simulink model "lane_following_AMPC"  (R2018b)
settings: Solver=VariableStepAuto  StartTime=0.0  StopTime=Duration  RelTol=1e-3
undefined symbols (not defined in the file or in its folder): Cf, Cr, Iz, lf, lr, m, rho, tau, Ts, v0, v_set
libraries: mpclib x1
settings Model: Creator=alberto  LastModifiedBy=alberto

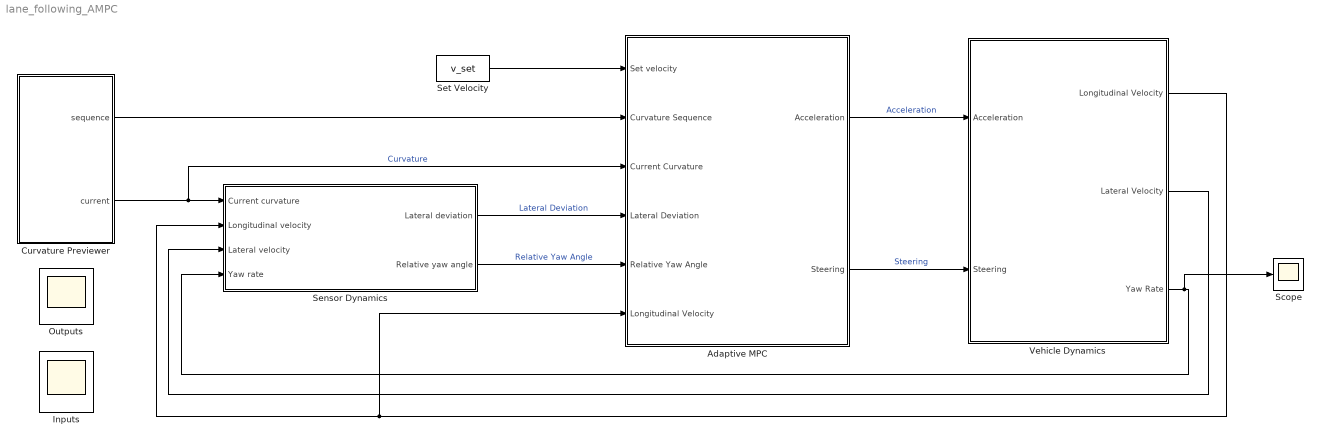
== system lane_following_AMPC ==
  Adaptive MPC : Subsystem  VariantControl=controller_type == 2
  Curvature Previewer : Subsystem  mask{signal=rho, ts=Ts, steps=25}
      mask prompts: signal "Signal name"; ts "Sampling time"; steps "Number of previewing steps"
      mask init:
      | ts = evalin('base',get_param(gcbh,'ts'));
      | signal = evalin('base',get_param(gcbh,'signal'));
      | steps = evalin('base',get_param(gcbh,'steps'));
      | data = mpc_previewer_maskinit(signal,ts);
      mask Display:
      | fprintf('Future\nsample\nextractor');
      | port_label('output', 1, 'seq')
      | port_label('output', 2, '@t')
  Inputs : Scope
      settings: Floating=on
  Outputs : Scope
      settings: Floating=on
  Scope : Scope
  Sensor Dynamics : Subsystem
  Set Velocity : Constant  Value=v_set
  Vehicle Dynamics : Subsystem
  wires:
  Curvature Previewer/2(current) -> Adaptive MPC/3(Current Curvature), Sensor Dynamics/1(Current curvature)  "Curvature"
  Sensor Dynamics/1(Lateral deviation) -> Adaptive MPC/4(Lateral Deviation)  "Lateral Deviation"
  Curvature Previewer/1(sequence) -> Adaptive MPC/2(Curvature Sequence)
  Sensor Dynamics/2(Relative yaw angle) -> Adaptive MPC/5(Relative Yaw Angle)  "Relative Yaw Angle"
  Adaptive MPC/2(" Steering") -> Vehicle Dynamics/2(Steering)  "Steering"
  Set Velocity/1 -> Adaptive MPC/1(Set velocity)
  Adaptive MPC/1(Acceleration) -> Vehicle Dynamics/1(Acceleration)  "Acceleration"
  Vehicle Dynamics/2(Lateral Velocity) -> Sensor Dynamics/3(Lateral velocity)
  Vehicle Dynamics/3(Yaw Rate) -> Scope/1, Sensor Dynamics/4(Yaw rate)
  Vehicle Dynamics/1(Longitudinal Velocity) -> Sensor Dynamics/2(Longitudinal velocity), Adaptive MPC/6(Longitudinal Velocity)

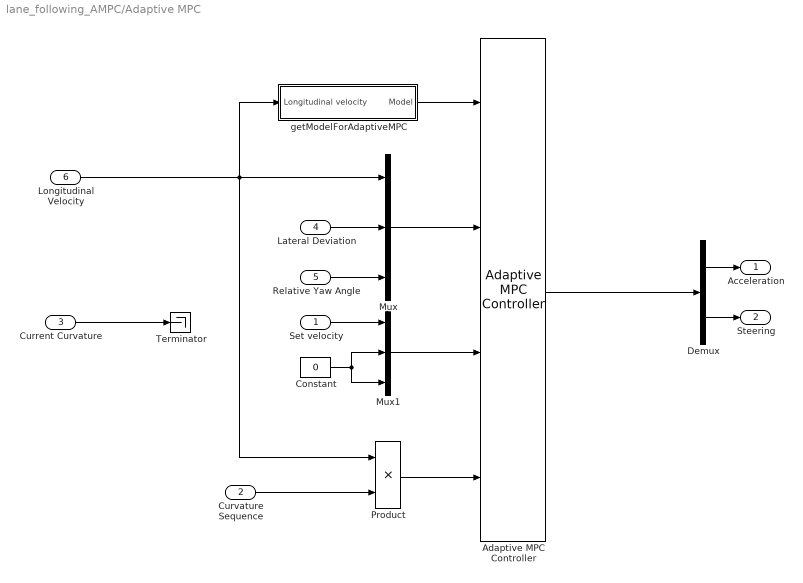
== system lane_following_AMPC/Adaptive MPC ==
  Set velocity : Inport
  Curvature Sequence : Inport  Port=2
  Current Curvature : Inport  Port=3
  Lateral Deviation : Inport  Port=4
  Relative Yaw Angle : Inport  Port=5
  Longitudinal Velocity : Inport  Port=6
  Adaptive MPC Controller : mpclib/Adaptive MPC Controller  SCDEnableBlockLinearizationSpecification=on  mpcobj=mpc1  enable_value=0  updateMPCinCallerWorkspace=on  md_inport=on  mv_inport=off  return_cost=off  return_mvseq=off  return_qpstatus=off  return_xseq=off  return_state=off  return_ovseq=off  state_inport=off  isltv_plant=off  umin_inport=off  umax_inport=off  ymin_inport=off  ymax_inport=off  cc_inport=off  ywt_inport=off  uwt_inport=off  duwt_inport=off  rhoeps_inport=off  uref_inport=off  BlockDataType=double  SampleTimeInherited=off  switch_inport=off
      settings: SourceProductName=Model Predictive Control Toolbox
  Constant : Constant  Value=0
  Demux : Demux  Outputs=2
  Mux : Mux  Inputs=3
  Mux1 : Mux  Inputs=3
  Product : Product
  Terminator : Terminator
  getModelForAdaptiveMPC : Subsystem
  Acceleration : Outport
  " Steering" : Outport  Port=2
  wires:
  Lateral Deviation/1 -> Mux/2
  Longitudinal Velocity/1 -> Product/1, Mux/1, getModelForAdaptiveMPC/1(Longitudinal velocity)
  Relative Yaw Angle/1 -> Mux/3
  Demux/2 -> " Steering"/1
  Set velocity/1 -> Mux1/1
  Demux/1 -> Acceleration/1
  Mux/1 -> Adaptive MPC Controller/2
  Mux1/1 -> Adaptive MPC Controller/3
  Constant/1 -> Mux1/3, Mux1/2
  Product/1 -> Adaptive MPC Controller/4
  getModelForAdaptiveMPC/1(Model) -> Adaptive MPC Controller/1
  Curvature Sequence/1 -> Product/2
  Current Curvature/1 -> Terminator/1
  Adaptive MPC Controller/1 -> Demux/1

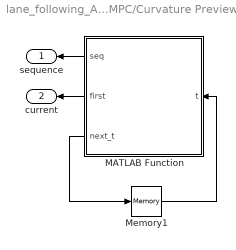
== system lane_following_AMPC/Curvature Previewer ==
  MATLAB Function : MATLAB Function  TreatAsAtomicUnit=on
  Memory1 : Memory  InheritSampleTime=on  LinearizeAsDelay=on
  sequence : Outport
  current : Outport  Port=2
  wires:
  MATLAB Function/1(seq) -> sequence/1
  MATLAB Function/2(first) -> current/1
  Memory1/1 -> MATLAB Function/1(t)
  MATLAB Function/3(next_t) -> Memory1/1

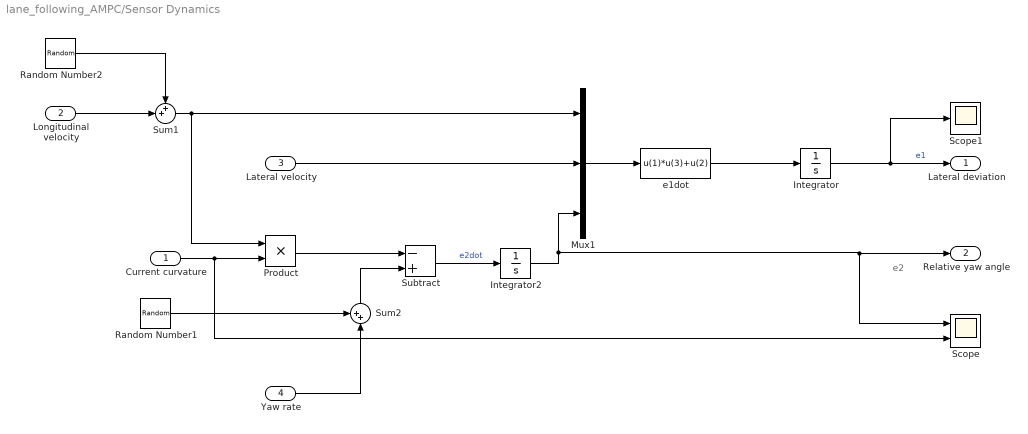
== system lane_following_AMPC/Sensor Dynamics ==
  note: e2
  Current curvature : Inport
  Longitudinal velocity : Inport  Port=2
  Lateral velocity : Inport  Port=3
  Yaw rate : Inport  Port=4
  Integrator : Integrator
  Integrator2 : Integrator
  Mux1 : Mux  Inputs=[1 1 1]
  Product : Product
  Random Number1 : RandomNumber  Variance=0.0003  SampleTime=Ts
  Random Number2 : RandomNumber  Variance=0.3  SampleTime=Ts
  Scope : Scope  NumInputPorts=2
  Scope1 : Scope
  Subtract : Sum  Inputs=-+
  Sum1 : Sum  Inputs=++|
  Sum2 : Sum  Inputs=++|
  e1dot : Fcn  Expr=u(1)*u(3)+u(2)
  Lateral deviation : Outport
  Relative yaw angle : Outport  Port=2
  wires:
  Mux1/1 -> e1dot/1
  Lateral velocity/1 -> Mux1/2
  Product/1 -> Subtract/1
  Subtract/1 -> Integrator2/1  "e2dot"
  Current curvature/1 -> Scope/2, Product/2
  Integrator/1 -> Scope1/1, Lateral deviation/1  "e1"
  Integrator2/1 -> Scope/1, Relative yaw angle/1, Mux1/3
  e1dot/1 -> Integrator/1
  Sum1/1 -> Product/1, Mux1/1
  Longitudinal velocity/1 -> Sum1/2
  Random Number2/1 -> Sum1/1
  Yaw rate/1 -> Sum2/2
  Random Number1/1 -> Sum2/1
  Sum2/1 -> Subtract/2

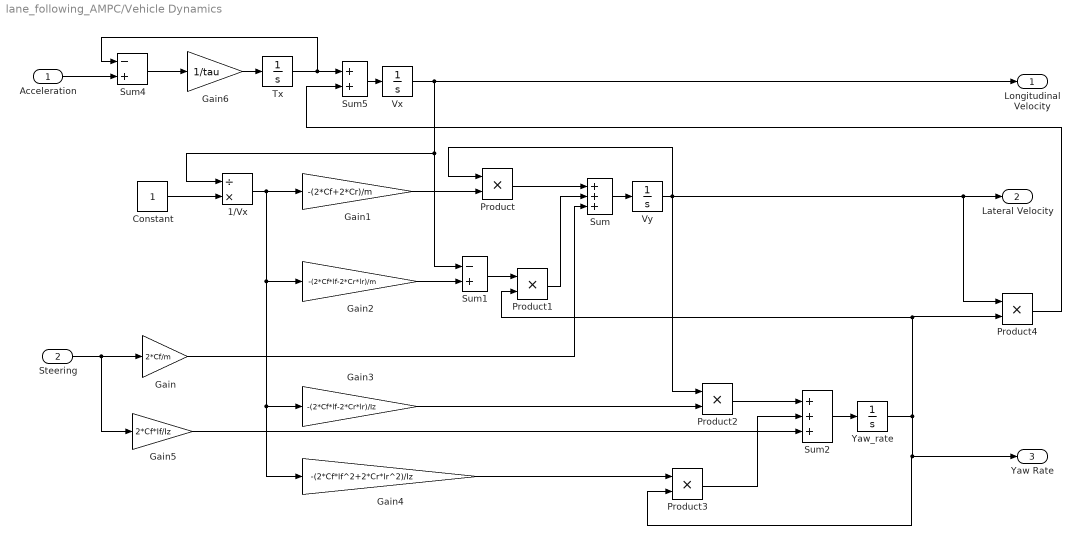
== system lane_following_AMPC/Vehicle Dynamics ==
  Acceleration : Inport
  Steering : Inport  Port=2
  1/Vx : Product  Inputs=/*
  Constant : Constant
  Gain : Gain  Gain=2*Cf/m
  Gain1 : Gain  Gain=-(2*Cf+2*Cr)/m
  Gain2 : Gain  Gain=-(2*Cf*lf-2*Cr*lr)/m
  Gain3 : Gain  Gain=-(2*Cf*lf-2*Cr*lr)/Iz
  Gain4 : Gain  Gain=-(2*Cf*lf^2+2*Cr*lr^2)/Iz
  Gain5 : Gain  Gain=2*Cf*lf/Iz
  Gain6 : Gain  Gain=1/tau
  Product{,1..4} (5 alike) : Product
  Sum : Sum  Inputs=+++
  Sum1 : Sum  Inputs=-+
  Sum2 : Sum  Inputs=+++
  Sum4 : Sum  Inputs=-+
  Sum5 : Sum
  Tx : Integrator
  Vx : Integrator  InitialCondition=v0
  Vy : Integrator
  "Yaw_rate " : Integrator
  Longitudinal Velocity : Outport
  Lateral Velocity : Outport  Port=2
  Yaw Rate : Outport  Port=3
  wires:
  Gain6/1 -> Tx/1
  Sum2/1 -> "Yaw_rate "/1
  Sum5/1 -> Vx/1
  Gain2/1 -> Sum1/2
  Gain4/1 -> Product3/1
  Constant/1 -> 1/Vx/2
  Gain3/1 -> Product2/2
  1/Vx/1 -> Gain4/1, Gain3/1, Gain2/1, Gain1/1
  Product2/1 -> Sum2/1
  Sum4/1 -> Gain6/1
  Acceleration/1 -> Sum4/2
  Tx/1 -> Sum5/1, Sum4/1
  Product3/1 -> Sum2/2
  Gain5/1 -> Sum2/3
  Product4/1 -> Sum5/2
  Sum1/1 -> Product1/1
  "Yaw_rate "/1 -> Yaw Rate/1, Product3/2, Product4/2, Product1/2
  Gain/1 -> Sum/3
  Steering/1 -> Gain/1, Gain5/1
  Gain1/1 -> Product/2
  Product/1 -> Sum/1
  Vy/1 -> Product/1, Lateral Velocity/1, Product4/1, Product2/1
  Sum/1 -> Vy/1
  Vx/1 -> Longitudinal Velocity/1, 1/Vx/1, Sum1/1
  Product1/1 -> Sum/2

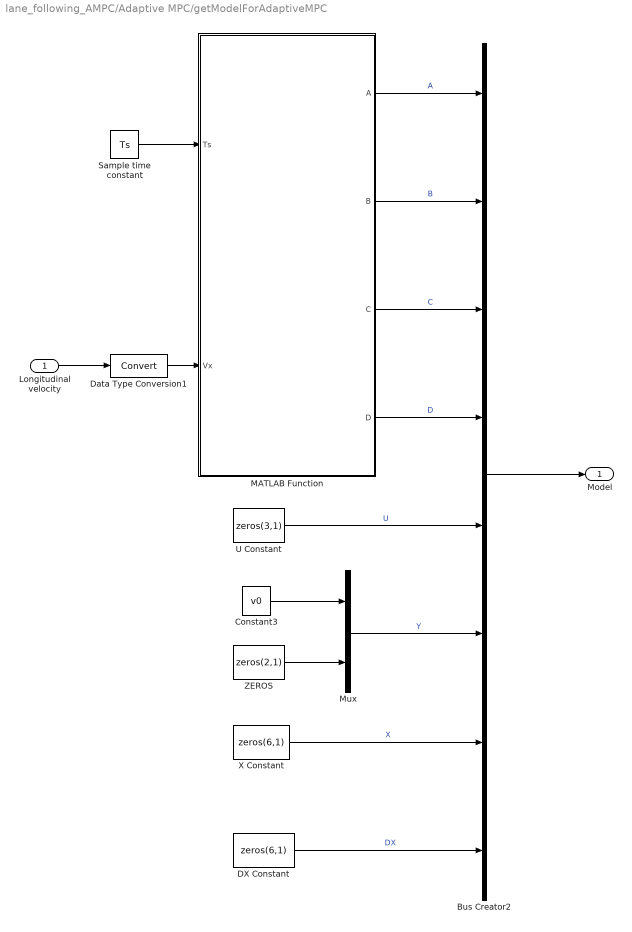
== system lane_following_AMPC/Adaptive MPC/getModelForAdaptiveMPC ==
  Longitudinal velocity : Inport
  Bus Creator2 : BusCreator  Inputs=8
  Constant3 : Constant  Value=v0
  DX Constant : Constant  Value=zeros(6,1)  VectorParams1D=off
  Data Type Conversion1 : DataTypeConversion
  MATLAB Function : MATLAB Function  TreatAsAtomicUnit=on
  Mux : Mux  Inputs=2
  Sample time constant : Constant  Value=Ts
  U Constant : Constant  Value=zeros(3,1)  VectorParams1D=off
  X Constant : Constant  Value=zeros(6,1)  VectorParams1D=off
  ZEROS : Constant  Value=zeros(2,1)  VectorParams1D=off
  Model : Outport
  wires:
  MATLAB Function/4(D) -> Bus Creator2/4  "D"
  X Constant/1 -> Bus Creator2/7  "X"
  Bus Creator2/1 -> Model/1
  Longitudinal velocity/1 -> Data Type Conversion1/1
  Mux/1 -> Bus Creator2/6  "Y"
  Sample time constant/1 -> MATLAB Function/1(Ts)
  MATLAB Function/1(A) -> Bus Creator2/1  "A"
  DX Constant/1 -> Bus Creator2/8  "DX"
  MATLAB Function/2(B) -> Bus Creator2/2  "B"
  MATLAB Function/3(C) -> Bus Creator2/3  "C"
  Data Type Conversion1/1 -> MATLAB Function/2(Vx)
  U Constant/1 -> Bus Creator2/5  "U"
  ZEROS/1 -> Mux/2
  Constant3/1 -> Mux/1

== matlab function lane_following_AMPC/Curvature Previewer/MATLAB Function ==
  settings: updateMethod=DISCRETE  sampleTime=ts
  data: data parameter; seq output; steps parameter; t input; first output; next_t output
function [seq,first,next_t] = fcn(data,steps,t)
%#codegen
[seq,first,next_t] = mpcblock_preview('md',data,steps,t);

== matlab function lane_following_AMPC/Adaptive MPC/getModelForAdaptiveMPC/MATLAB Function ==
  data: Ts input; A output; Vx input; B output; C output; D output
  function [A,B,C,D] = getAdaptiveMPCModel(Ts,Vx)
% Get discrete state-space model for Adaptive MPC with sample time Ts.
% Called by the "Lane Keeping Assist System" Block.

% Inputs:
%   Ts:               mask variable for sample time
%   Vx:               mask inport for longitudinal velocity
%   Curvature:        mask inport for curvature
%   lastU:            last MV value for MPC
%   measuredY:        mo value for MPC
%   Ag,Bg,Cg:         continuous or discrete vehicle model with sample time Ts              
% Outputs:
%   A,B,C,D:          discrete time model for adaptive MPC

%   Author: Meng Xia, Rong Chen
%   Copyright 2017-2018 The MathWorks, Inc.

m = 1575; % Mass of car
Iz = 2875; % Moment of inertia about Z axis
lf = 1.2; % Distance between Center of Gravity and Front axle 
lr = 1.6; % Distance between Center of Gravity and Rear axle
Cf = 19000; % Cornering stiffness of the front tires (N/rad)
Cr = 33000; % Cornering stiffness of the rear tires (N/rad).
tau = 0.2; % Time constant

a1 = -(2*Cf+2*Cr)/m/Vx;
a2 = -(2*Cf*lf-2*Cr*lr)/m/Vx - Vx;
a3 = -(2*Cf*lf-2*Cr*lr)/Iz/Vx;
a4 = -(2*Cf*lf^2+2*Cr*lr^2)/Iz/Vx;
b1 = 2*Cf/m;
b2 = 2*Cf*lf/Iz;

% Specify the vehicle model matrices with states [vy,phidot].
Ag = [a1,a2;a3,a4];
Bg = [b1;b2];
Cg = eye(2);
% Discrete MPC model
[A,B,C,D] = LaneFollowingGetModelForAMPC(Ts,Vx,Ag,Bg,Cg);
